simulink model "anti_windup"  (R2016a)
settings: Solver=ode45  StartTime=0.0  StopTime=20.0  RelTol=1e-3
undefined symbols (not defined in the file or in its folder): i
settings Model: Creator=kjartan  LastModifiedBy=kjartan
settings DataIOCC: LimitDataPoints=on  SaveFormat=Array
settings DebuggingCC: SolverPrmCheckMsg=warning
settings HardwareCC: ProdBitPerPointer=32  ProdLargestAtomicFloat=None  ProdIntDivRoundTo=Undefined  ProdEndianess=Unspecified  ProdWordSize=32  ProdHWDeviceType=32-bit Generic
settings ModelReferenceCC: PropagateSignalLabelsOutOfModel=off
settings ConfigComp: CovModelRefEnable=Off  CovSFcnEnable=off

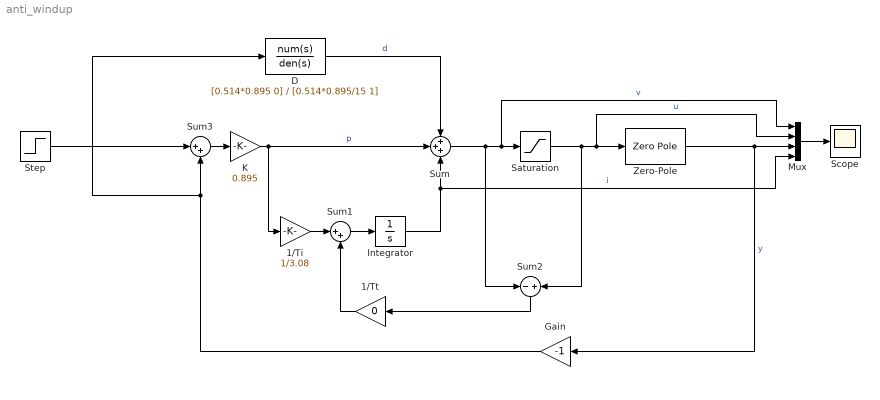
== system anti_windup ==
  1/Ti : Gain  Gain=1/3.08
  1/Tt : Gain  Gain=0
  D : TransferFcn  Numerator=[0.514*0.895 0]  Denominator=[0.514*0.895/15 1]
  Gain : Gain  Gain=-1
  Integrator : Integrator
  K : Gain  Gain=0.895
  Mux : Mux
  Saturation : Saturate  UpperLimit=0.3  LowerLimit=-0.3
  Scope : Scope
  Step : Step  SampleTime=0
  Sum : Sum  Inputs=+++
  Sum1 : Sum  Inputs=|++
  Sum2 : Sum  Inputs=-|+
  Sum3 : Sum  Inputs=|++
  Zero-Pole : ZeroPole  Zeros=[-3]  Poles=[0 -2 -1+2*i, -1-2*i]  Gain=[5]
  wires:
  Saturation/1 -> Sum2/2, Mux/2, Zero-Pole/1  "u"
  Sum/1 -> Sum2/1, Mux/1, Saturation/1  "v"
  D/1 -> Sum/1  "d"
  K/1 -> 1/Ti/1, Sum/2  "p"
  1/Ti/1 -> Sum1/1
  Sum1/1 -> Integrator/1
  Integrator/1 -> Mux/4, Sum/3  "i"
  Sum2/1 -> 1/Tt/1
  1/Tt/1 -> Sum1/2
  Zero-Pole/1 -> Gain/1, Mux/3  "y"
  Gain/1 -> Sum3/2, D/1
  Step/1 -> Sum3/1
  Sum3/1 -> K/1
  Mux/1 -> Scope/1
